simulink model "simulare"  (R2023b)
settings: Solver=VariableStepAuto  StartTime=0.0  StopTime=10.0  RelTol=1e-3
settings Model: Creator=Lenovo  LastModifiedBy=Lenovo

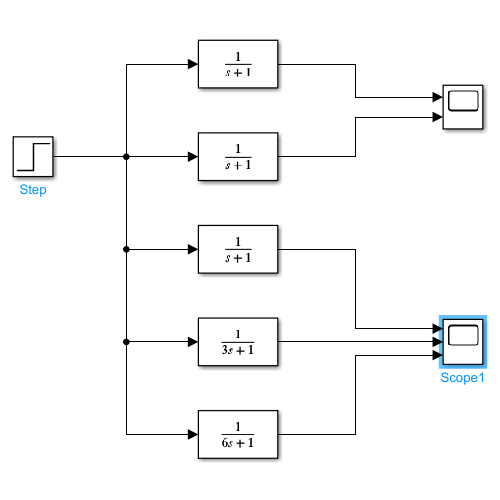
[thumbnail: Simulink's stored preview of the top-level diagram]
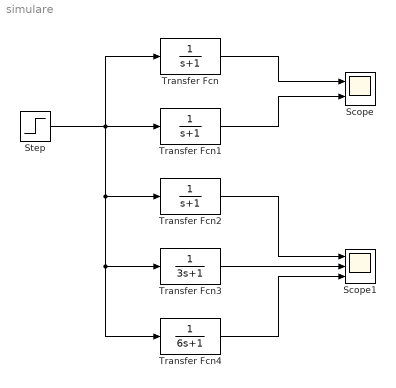
== system simulare ==
  Scope : Scope  NumInputPorts=2
  Scope1 : Scope  NumInputPorts=3
  Step : Step  SampleTime=0
  Transfer Fcn : TransferFcn  Denominator=[1 1]
  Transfer Fcn1 : TransferFcn  Denominator=[1 1]
  Transfer Fcn2 : TransferFcn  Denominator=[1 1]
  Transfer Fcn3 : TransferFcn  Denominator=[3 1]
  Transfer Fcn4 : TransferFcn  Denominator=[6 1]
  wires:
  Step/1 -> Transfer Fcn4/1, Transfer Fcn3/1, Transfer Fcn2/1, Transfer Fcn/1, Transfer Fcn1/1
  Transfer Fcn/1 -> Scope/1
  Transfer Fcn1/1 -> Scope/2
  Transfer Fcn2/1 -> Scope1/1
  Transfer Fcn3/1 -> Scope1/2
  Transfer Fcn4/1 -> Scope1/3
